simulink model "untitled"  (R2015a)
settings: Solver=ode45  StartTime=0.0  StopTime=1  RelTol=1e-3
libraries: powerlib x11
settings Model: Creator=MBK  LastModifiedBy=MBK

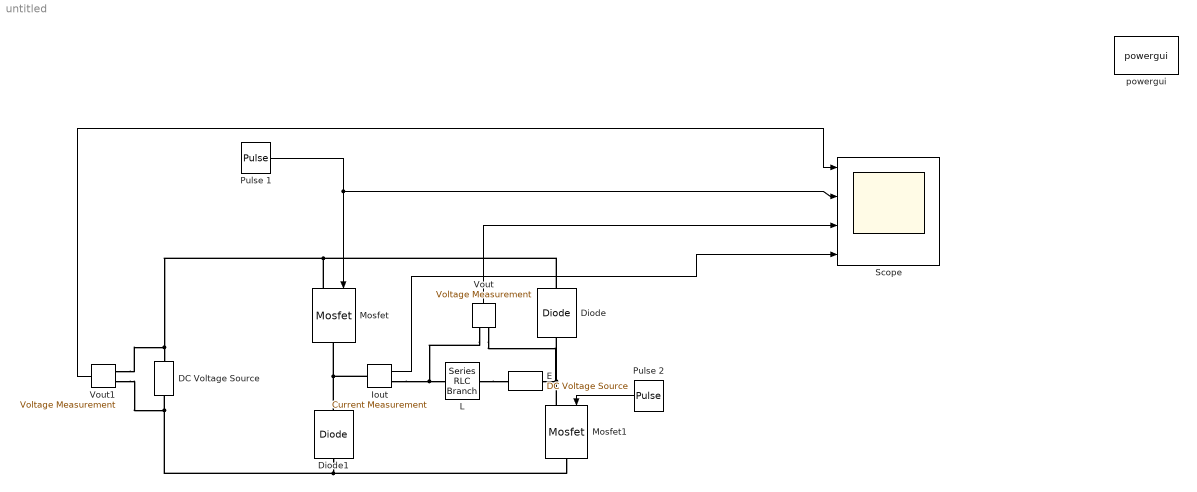
== system untitled ==
  DC Voltage Source : powerlib/Electrical Sources/DC Voltage Source  Amplitude=240  Measurements=None
  Diode : powerlib/Power Electronics/Diode  Ron=0.001  Lon=0  Vf=0.8  IC=0  UseSnubber=off  Rs=500  Cs=250e-9  Measurements=off
  Diode1 : powerlib/Power Electronics/Diode  Ron=0.001  Lon=0  Vf=0.8  IC=0  UseSnubber=off  Rs=500  Cs=250e-9  Measurements=off
  E : powerlib/Electrical Sources/DC Voltage Source  Amplitude=12  Measurements=None
  Iout : powerlib/Measurements/Current Measurement  PhasorSimulation=off  OutputType=Complex  PSBequivalent=0
  L : powerlib/Elements/Series RLC Branch  LConnTagsString=__new0  RConnTagsString=__new0  BranchType=RL  Resistance=10  Inductance=100e-3  SetiL0=off  InitialCurrent=0  Capacitance=1e-6  Setx0=off  InitialVoltage=0  Measurements=None
  Mosfet : powerlib/Power Electronics/Mosfet  Ron=0.1  Lon=0  Rd=0.01  Vfd=0  IC=0  Rs=1e5  Cs=inf  Measurements=off
  Mosfet1 : powerlib/Power Electronics/Mosfet  Ron=0.1  Lon=0  Rd=0.01  Vfd=0  IC=0  Rs=1e5  Cs=inf  Measurements=off
  Pulse 1 : DiscretePulseGenerator  PulseType=Time based  Amplitude=10  Period=0.02  PulseWidth=80
  Pulse 2 : DiscretePulseGenerator  PulseType=Time based  Amplitude=10  Period=0.02  PulseWidth=80
  Scope : Scope  NumInputPorts=4
      settings: ShowLegends=on  YMin=-5~-5~-5~-5  YMax=5~5~5~5
  Vout : powerlib/Measurements/Voltage Measurement  PhasorSimulation=off  OutputType=Complex  PSBequivalent=0
  Vout1 : powerlib/Measurements/Voltage Measurement  PhasorSimulation=off  OutputType=Complex  PSBequivalent=0
  powergui : powerlib/powergui  Priority=1  SimulationMode=Continuous  SolverType=Tustin/Backward Euler (TBE)  SampleTime=50e-6  frequency=60  SPID=off  DisableSnubberDevices=off  DisableRonSwitches=off  DisableVfSwitches=off  SwTol=0  DisplayEquations=off  Interpol=off  methode=off  Ts=100  FunctionMessages=off  echomessages=off  HookPort=off  EnableUseOfTLC=off  x0status=blocks  frequencyindice=0  Pbase=100e6  ErrMax=1e-4  Iterations=50  UnitsV=kV  UnitsW=MW  buscounter=0  RestoreLinks=warning  ResistiveCurrentMeasurement=off  Frange=[0:2:500]  Ylog=off  Xlog=on  ShowGrid=off  save=off  variable=ZData  structure=0  ZoomFFT=off  StartTime=0.0  cycles=1  DisplayStyle=1  fundamental=60  FreqAxis=off  MaxFrequency=1000  frequencyindicesteady=1  RmsSteady=1  display=off
  wires:
  Vout1/1 -> Scope/1
  Pulse 1/1 -> Scope/2, Mosfet/1
  Pulse 2/1 -> Mosfet1/1
  Vout/1 -> Scope/3
  Iout/1 -> Scope/4
  connections:
  Vout1/LConn2 -- Mosfet1/RConn1 -- Diode1/LConn1 -- DC Voltage Source/LConn1
  Vout1/LConn1 -- Diode/RConn1 -- Mosfet/LConn1 -- DC Voltage Source/RConn1
  L/RConn1 -- E/RConn1
  Diode1/RConn1 -- Iout/LConn1 -- Mosfet/RConn1
  Mosfet1/LConn1 -- Diode/LConn1 -- Vout/LConn2 -- E/LConn1
  Iout/RConn1 -- Vout/LConn1 -- L/LConn1
